simulink model "SmartAccess_20221026"  (R2022b)
settings: Solver=FixedStepDiscrete  StartTime=0.0  StopTime=10.0  RelTol=1e-3
undefined symbols (not defined in the file): AppPassthroughCommunicationOutputExternal, ApproachDetected, BasicUserInteractionFramework, GenericBackendMCPReceptions, GenericTelematicMCPReception, KeyPositionDetected, KeyProximityDetected, KeySearchRequest, KeyTrajectoryDetected, RequestDisplayCheckControl, RequestKeyPositionTracking, RequestKeyProximityTracking, RequestZa03ParkingandRemote, RequestZa06KlimaBasis, SendSmartAccessBackendData, SmartAccessEventNofitication, SmartAccessEventNotification, SmartAccessManageKey, SmartAccessTrackKey, SmartAccessVehicleUIControlAndStatus, StatusVehicleOccupantInformation, StopKeyPositionTracking, UpdateSmartAccessBackendData
settings Model: Creator=lcx19  LastModifiedBy=lcx19

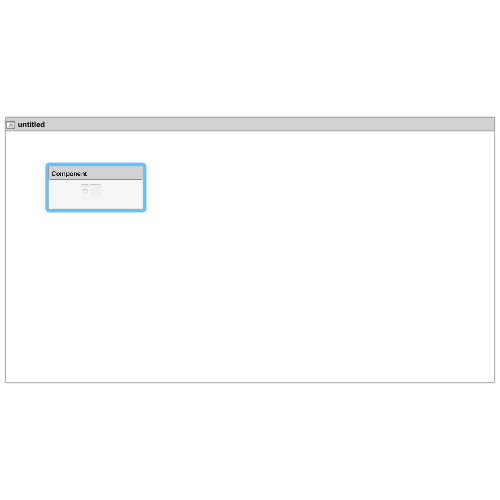
[thumbnail: Simulink's stored preview of the top-level diagram]
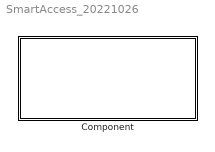
== system SmartAccess_20221026 ==
  Component : Subsystem
      settings: PortSchema="{\"entries\":[{\"content\":{\"headerSize\":26,\"margin\":15,\"minimumSpacing\":25,\"sides\":[{\"content\":{\"connectorIds\":[]},\"type\":\"ConnectorPlacement.EquallySpacedRectSide\",\"uuid\":\"a28210fe-8bcc-4966-9def-b490f12f7165\"},{\"content\":{\"connectorIds\":[],\"side\":\"RIGHT\"},\"type\":\"ConnectorPlacement.EquallySpacedRectSide\",\"uuid\":\"9429c510-dad9-436c-8408-75f9033cfc3b\"},{\"content\":{\"connectorIds\":[],\"side\":\"TOP\"},\"type\":\"ConnectorPlacement.EquallySpacedRectSide\",\"uuid\":\"a13e5907-bdbb-46b5-9334-9875d9723f49\"}]},\"type\":\"ConnectorPlacement.EquallySpacedConnector\",\"uuid\":\"ba0b5127-fa18-4541-84db-e1fe9f0ba6eb\"}],\"packageUris\":[\"http://schema.mathworks.com/mf0/Connector/R2020b\"],\"version\":\"1.0\"}"

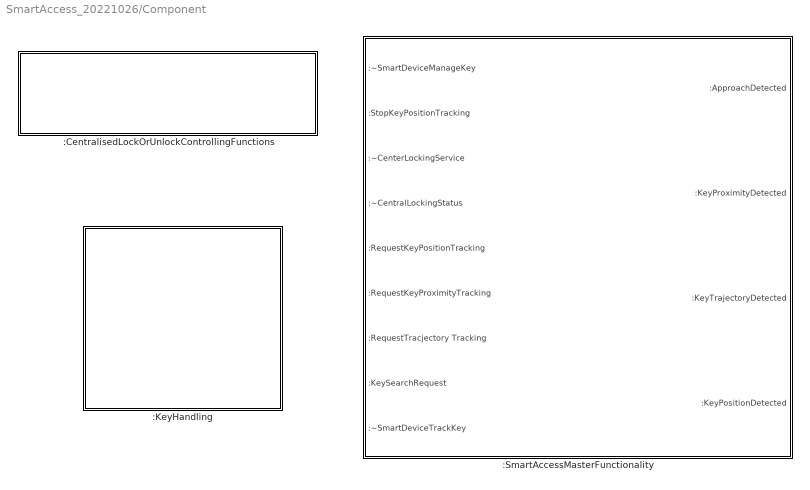
== system SmartAccess_20221026/Component ==
  :CentralisedLockOrUnlockControllingFunctions : Subsystem
      settings: PortSchema="{\"entries\":[{\"content\":{\"headerSize\":26,\"margin\":15,\"minimumSpacing\":25,\"sides\":[{\"content\":{\"connectorIds\":[]},\"type\":\"ConnectorPlacement.EquallySpacedRectSide\",\"uuid\":\"a28210fe-8bcc-4966-9def-b490f12f7165\"},{\"content\":{\"connectorIds\":[],\"side\":\"RIGHT\"},\"type\":\"ConnectorPlacement.EquallySpacedRectSide\",\"uuid\":\"9429c510-dad9-436c-8408-75f9033cfc3b\"},{\"content\":{\"connectorIds\":[],\"side\":\"TOP\"},\"type\":\"ConnectorPlacement.EquallySpacedRectSide\",\"uuid\":\"a13e5907-bdbb-46b5-9334-9875d9723f49\"}]},\"type\":\"ConnectorPlacement.EquallySpacedConnector\",\"uuid\":\"ba0b5127-fa18-4541-84db-e1fe9f0ba6eb\"}],\"packageUris\":[\"http://schema.mathworks.com/mf0/Connector/R2020b\"],\"version\":\"1.0\"}"
  :KeyHandling : Subsystem
      settings: PortSchema="{\"entries\":[{\"content\":{\"headerSize\":26,\"margin\":15,\"minimumSpacing\":25,\"sides\":[{\"content\":{\"connectorIds\":[]},\"type\":\"ConnectorPlacement.EquallySpacedRectSide\",\"uuid\":\"a28210fe-8bcc-4966-9def-b490f12f7165\"},{\"content\":{\"connectorIds\":[],\"side\":\"RIGHT\"},\"type\":\"ConnectorPlacement.EquallySpacedRectSide\",\"uuid\":\"9429c510-dad9-436c-8408-75f9033cfc3b\"},{\"content\":{\"connectorIds\":[],\"side\":\"TOP\"},\"type\":\"ConnectorPlacement.EquallySpacedRectSide\",\"uuid\":\"a13e5907-bdbb-46b5-9334-9875d9723f49\"}]},\"type\":\"ConnectorPlacement.EquallySpacedConnector\",\"uuid\":\"ba0b5127-fa18-4541-84db-e1fe9f0ba6eb\"}],\"packageUris\":[\"http://schema.mathworks.com/mf0/Connector/R2020b\"],\"version\":\"1.0\"}"
  :SmartAccessMasterFunctionality : Subsystem
      settings: PortSchema="{\"entries\":[{\"content\":{\"headerSize\":26,\"margin\":15,\"minimumSpacing\":25,\"sides\":[{\"content\":{\"connectorIds\":[\"In1\",\"In2\",\"Out1\",\"In3\",\"In4\",\"In5\",\"In6\",\"In7\",\"In8\"]},\"type\":\"ConnectorPlacement.EquallySpacedRectSide\",\"uuid\":\"a28210fe-8bcc-4966-9def-b490f12f7165\"},{\"content\":{\"connectorIds\":[\"Out2\",\"Out3\",\"Out4\",\"Out5\"],\"side\":\"RIGHT\"},\"type\":\"ConnectorPlacement.EquallySpacedRectSide\",\"uuid\":\"9429c510-dad9-436c-8408-75f9033cfc3b\"},{\"content\":{\"connectorIds\":[],\"side\":\"TOP\"},\"type\":\"ConnectorPlacement.EquallySpacedRectSide\",\"uuid\":\"a13e5907-bdbb-46b5-9334-9875d9723f49\"}]},\"type\":\"ConnectorPlacement.EquallySpacedConnector\",\"uuid\":\"ba0b5127-fa18-4541-84db-e1fe9f0ba6eb\"}],\"packageUris\":[\"http://schema.mathworks.com/mf0/Connector/R2020b\"],\"version\":\"1.0\"}"

== system SmartAccess_20221026/Component/:CentralisedLockOrUnlockControllingFunctions ==

== system SmartAccess_20221026/Component/:KeyHandling ==

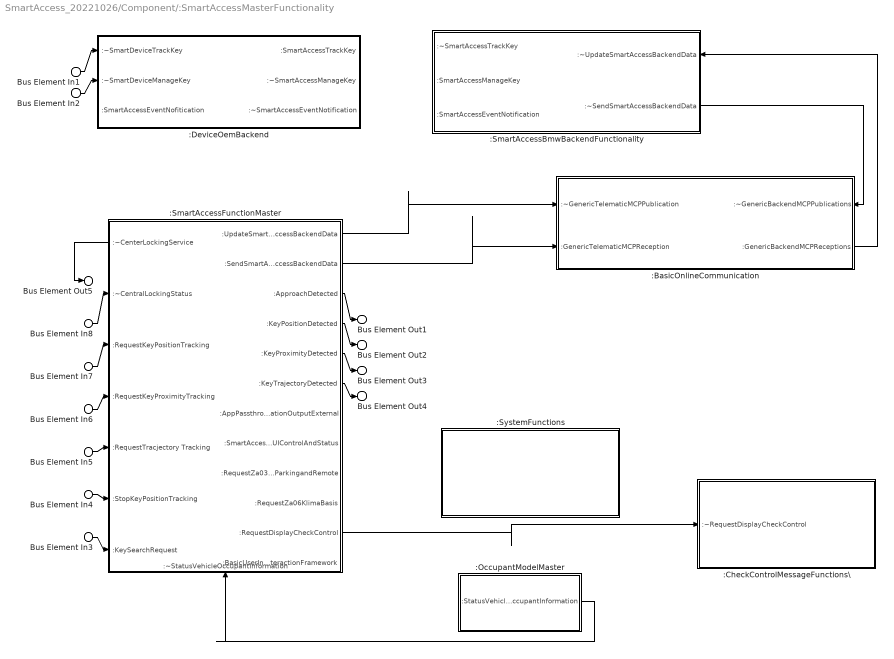
== system SmartAccess_20221026/Component/:SmartAccessMasterFunctionality ==
  Bus Element In2 : Inport  PortName=:~SmartDeviceManageKey
  Bus Element In4 : Inport  Port=2  PortName=:StopKeyPositionTracking
  Bus Element In8 : Inport  Port=3  PortName=:~CentralLockingStatus
  Bus Element In7 : Inport  Port=4  PortName=:RequestKeyPositionTracking
  Bus Element In6 : Inport  Port=5  PortName=:RequestKeyProximityTracking
  Bus Element In5 : Inport  Port=6  PortName=:RequestTracjectory Tracking
  Bus Element In3 : Inport  Port=7  PortName=:KeySearchRequest
  Bus Element In1 : Inport  Port=8  PortName=:~SmartDeviceTrackKey
  :BasicOnlineCommunication : Subsystem
      settings: PortSchema="{\"entries\":[{\"content\":{\"headerSize\":26,\"margin\":15,\"minimumSpacing\":25,\"sides\":[{\"content\":{\"connectorIds\":[\"In1\",\"In2\"]},\"type\":\"ConnectorPlacement.EquallySpacedRectSide\",\"uuid\":\"a28210fe-8bcc-4966-9def-b490f12f7165\"},{\"content\":{\"connectorIds\":[\"In3\",\"Out1\"],\"side\":\"RIGHT\"},\"type\":\"ConnectorPlacement.EquallySpacedRectSide\",\"uuid\":\"9429c510-dad9-436c-8408-75f9033cfc3b\"},{\"content\":{\"connectorIds\":[],\"side\":\"TOP\"},\"type\":\"ConnectorPlacement.EquallySpacedRectSide\",\"uuid\":\"a13e5907-bdbb-46b5-9334-9875d9723f49\"}]},\"type\":\"ConnectorPlacement.EquallySpacedConnector\",\"uuid\":\"ba0b5127-fa18-4541-84db-e1fe9f0ba6eb\"}],\"packageUris\":[\"http://schema.mathworks.com/mf0/Connector/R2020b\"],\"version\":\"1.0\"}"
  :CheckControlMessageFunctions\ : Subsystem
      settings: PortSchema="{\"entries\":[{\"content\":{\"headerSize\":26,\"margin\":15,\"minimumSpacing\":25,\"sides\":[{\"content\":{\"connectorIds\":[\"In1\"]},\"type\":\"ConnectorPlacement.EquallySpacedRectSide\",\"uuid\":\"a28210fe-8bcc-4966-9def-b490f12f7165\"},{\"content\":{\"connectorIds\":[],\"side\":\"RIGHT\"},\"type\":\"ConnectorPlacement.EquallySpacedRectSide\",\"uuid\":\"9429c510-dad9-436c-8408-75f9033cfc3b\"},{\"content\":{\"connectorIds\":[],\"side\":\"TOP\"},\"type\":\"ConnectorPlacement.EquallySpacedRectSide\",\"uuid\":\"a13e5907-bdbb-46b5-9334-9875d9723f49\"}]},\"type\":\"ConnectorPlacement.EquallySpacedConnector\",\"uuid\":\"ba0b5127-fa18-4541-84db-e1fe9f0ba6eb\"}],\"packageUris\":[\"http://schema.mathworks.com/mf0/Connector/R2020b\"],\"version\":\"1.0\"}"
  :DeviceOemBackend : Subsystem
      settings: PortSchema="{\"entries\":[{\"content\":{\"headerSize\":26,\"margin\":15,\"minimumSpacing\":25,\"sides\":[{\"content\":{\"connectorIds\":[\"In2\",\"In3\",\"In4\"]},\"type\":\"ConnectorPlacement.EquallySpacedRectSide\",\"uuid\":\"a28210fe-8bcc-4966-9def-b490f12f7165\"},{\"content\":{\"connectorIds\":[\"Out1\",\"Out2\",\"In1\"],\"side\":\"RIGHT\"},\"type\":\"ConnectorPlacement.EquallySpacedRectSide\",\"uuid\":\"9429c510-dad9-436c-8408-75f9033cfc3b\"},{\"content\":{\"connectorIds\":[],\"side\":\"TOP\"},\"type\":\"ConnectorPlacement.EquallySpacedRectSide\",\"uuid\":\"a13e5907-bdbb-46b5-9334-9875d9723f49\"}]},\"type\":\"ConnectorPlacement.EquallySpacedConnector\",\"uuid\":\"ba0b5127-fa18-4541-84db-e1fe9f0ba6eb\"}],\"packageUris\":[\"http://schema.mathworks.com/mf0/Connector/R2020b\"],\"version\":\"1.0\"}"
  :OccupantModelMaster : Subsystem
      settings: PortSchema="{\"entries\":[{\"content\":{\"headerSize\":26,\"margin\":15,\"minimumSpacing\":25,\"sides\":[{\"content\":{\"connectorIds\":[]},\"type\":\"ConnectorPlacement.EquallySpacedRectSide\",\"uuid\":\"a28210fe-8bcc-4966-9def-b490f12f7165\"},{\"content\":{\"connectorIds\":[\"Out1\"],\"side\":\"RIGHT\"},\"type\":\"ConnectorPlacement.EquallySpacedRectSide\",\"uuid\":\"9429c510-dad9-436c-8408-75f9033cfc3b\"},{\"content\":{\"connectorIds\":[],\"side\":\"TOP\"},\"type\":\"ConnectorPlacement.EquallySpacedRectSide\",\"uuid\":\"a13e5907-bdbb-46b5-9334-9875d9723f49\"}]},\"type\":\"ConnectorPlacement.EquallySpacedConnector\",\"uuid\":\"ba0b5127-fa18-4541-84db-e1fe9f0ba6eb\"}],\"packageUris\":[\"http://schema.mathworks.com/mf0/Connector/R2020b\"],\"version\":\"1.0\"}"
  :SmartAccessBmwBackendFunctionality : Subsystem
      settings: PortSchema="{\"entries\":[{\"content\":{\"headerSize\":26,\"margin\":15,\"minimumSpacing\":25,\"sides\":[{\"content\":{\"connectorIds\":[\"In2\",\"In3\",\"Out2\"]},\"type\":\"ConnectorPlacement.EquallySpacedRectSide\",\"uuid\":\"a28210fe-8bcc-4966-9def-b490f12f7165\"},{\"content\":{\"connectorIds\":[\"In1\",\"Out1\"],\"side\":\"RIGHT\"},\"type\":\"ConnectorPlacement.EquallySpacedRectSide\",\"uuid\":\"9429c510-dad9-436c-8408-75f9033cfc3b\"},{\"content\":{\"connectorIds\":[],\"side\":\"TOP\"},\"type\":\"ConnectorPlacement.EquallySpacedRectSide\",\"uuid\":\"a13e5907-bdbb-46b5-9334-9875d9723f49\"}]},\"type\":\"ConnectorPlacement.EquallySpacedConnector\",\"uuid\":\"ba0b5127-fa18-4541-84db-e1fe9f0ba6eb\"}],\"packageUris\":[\"http://schema.mathworks.com/mf0/Connector/R2020b\"],\"version\":\"1.0\"}"
  :SmartAccessFunctionMaster : Subsystem
      settings: PortSchema="{\"entries\":[{\"content\":{\"headerSize\":26,\"margin\":15,\"minimumSpacing\":25,\"sides\":[{\"content\":{\"connectorIds\":[\"Out1\",\"In1\",\"In2\",\"In3\",\"In4\",\"In5\",\"In6\"]},\"type\":\"ConnectorPlacement.EquallySpacedRectSide\",\"uuid\":\"a28210fe-8bcc-4966-9def-b490f12f7165\"},{\"content\":{\"connectorIds\":[\"Out2\",\"Out3\",\"Out4\",\"Out5\",\"Out6\",\"Out7\",\"Out8\",\"Out9\",\"Out10\",\"Out11\",\"Out12\",\"Out13\"],\"side\":\"RIGHT\"},\"type\":\"ConnectorPlacement.EquallySpacedRectSide\",\"uuid\":\"9429c510-dad9-436c-8408-75f9033cfc3b\"},{\"content\":{\"connectorIds\":[],\"side\":\"TOP\"},\"type\":\"ConnectorPlacement.EquallySpacedRectSide\",\"uuid\":\"a13e5907-bdbb-46b5-9334-9875d9723f49\"},{\"content\":{\"connectorIds\":[\"In7\"],\"side\":\"BOTTOM\"},\"type\":\"ConnectorPlacement.EquallySpacedRectSide\",\"uuid\":\"de40a1c8-ef0d-4a2a-ba46-2e2a24800d7b\"}]},\"type\":\"ConnectorPlacement.EquallySpacedConnector\",\"uuid\":\"ba0b5127-fa18-4541-84db-e1fe9f0ba6eb\"}],\"packageUris\":[\"http://schema.mathworks.com/mf0/Connector/R2020b\"],\"version\":\"1.0\"}"
  :SystemFunctions : Subsystem
      settings: PortSchema="{\"entries\":[{\"content\":{\"headerSize\":26,\"margin\":15,\"minimumSpacing\":25,\"sides\":[{\"content\":{\"connectorIds\":[]},\"type\":\"ConnectorPlacement.EquallySpacedRectSide\",\"uuid\":\"a28210fe-8bcc-4966-9def-b490f12f7165\"},{\"content\":{\"connectorIds\":[],\"side\":\"RIGHT\"},\"type\":\"ConnectorPlacement.EquallySpacedRectSide\",\"uuid\":\"9429c510-dad9-436c-8408-75f9033cfc3b\"},{\"content\":{\"connectorIds\":[],\"side\":\"TOP\"},\"type\":\"ConnectorPlacement.EquallySpacedRectSide\",\"uuid\":\"a13e5907-bdbb-46b5-9334-9875d9723f49\"}]},\"type\":\"ConnectorPlacement.EquallySpacedConnector\",\"uuid\":\"ba0b5127-fa18-4541-84db-e1fe9f0ba6eb\"}],\"packageUris\":[\"http://schema.mathworks.com/mf0/Connector/R2020b\"],\"version\":\"1.0\"}"
  Bus Element Out5 : Outport  PortName=:~CenterLockingService
  Bus Element Out1 : Outport  Port=2  PortName=:ApproachDetected
  Bus Element Out3 : Outport  Port=3  PortName=:KeyProximityDetected
  Bus Element Out4 : Outport  Port=4  PortName=:KeyTrajectoryDetected
  Bus Element Out2 : Outport  Port=5  PortName=:KeyPositionDetected
  wires:
  Bus Element In1/1 -> :DeviceOemBackend/2(:~SmartDeviceTrackKey)
  Bus Element In2/1 -> :DeviceOemBackend/3(:~SmartDeviceManageKey)
  :SmartAccessBmwBackendFunctionality/1(:~SendSmartAccessBackendData) -> :BasicOnlineCommunication/3(:~GenericBackendMCPPublications)
  :BasicOnlineCommunication/1(:GenericBackendMCPReceptions) -> :SmartAccessBmwBackendFunctionality/1(:~UpdateSmartAccessBackendData)
  :SmartAccessFunctionMaster/2(:UpdateSmartAccessBackendData) -> :BasicOnlineCommunication/1(:~GenericTelematicMCPPublication)
  :SmartAccessFunctionMaster/3(:SendSmartAccessBackendData) -> :BasicOnlineCommunication/2(:GenericTelematicMCPReception)
  :SmartAccessFunctionMaster/4(:ApproachDetected) -> Bus Element Out1/1
  :SmartAccessFunctionMaster/5(:KeyPositionDetected) -> Bus Element Out2/1
  :SmartAccessFunctionMaster/6(:KeyProximityDetected) -> Bus Element Out3/1
  :SmartAccessFunctionMaster/7(:KeyTrajectoryDetected) -> Bus Element Out4/1
  :SmartAccessFunctionMaster/12(:RequestDisplayCheckControl) -> :CheckControlMessageFunctions\/1(:~RequestDisplayCheckControl)
  :OccupantModelMaster/1(:StatusVehicleOccupantInformation) -> :SmartAccessFunctionMaster/7(:~StatusVehicleOccupantInformation)
  Bus Element In3/1 -> :SmartAccessFunctionMaster/6(:KeySearchRequest)
  Bus Element In4/1 -> :SmartAccessFunctionMaster/5(:StopKeyPositionTracking)
  Bus Element In5/1 -> :SmartAccessFunctionMaster/4(:RequestTracjectory Tracking)
  :SmartAccessFunctionMaster/1(:~CenterLockingService) -> Bus Element Out5/1
  Bus Element In6/1 -> :SmartAccessFunctionMaster/3(:RequestKeyProximityTracking)
  Bus Element In7/1 -> :SmartAccessFunctionMaster/2(:RequestKeyPositionTracking)
  Bus Element In8/1 -> :SmartAccessFunctionMaster/1(:~CentralLockingStatus)

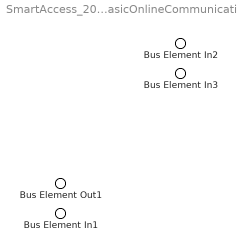
== system SmartAccess_20221026/Component/:SmartAccessMasterFunctionality/:BasicOnlineCommunication ==
  Bus Element In2 : Inport  PortName=:~GenericTelematicMCPPublication
  Bus Element In3 : Inport  Port=2  PortName=:GenericTelematicMCPReception
  Bus Element In1 : Inport  Port=3  PortName=:~GenericBackendMCPPublications
  Bus Element Out1 : Outport  PortName=:GenericBackendMCPReceptions

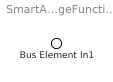
== system SmartAccess_20221026/Component/:SmartAccessMasterFunctionality/:CheckControlMessageFunctions\ ==
  Bus Element In1 : Inport  PortName=:~RequestDisplayCheckControl

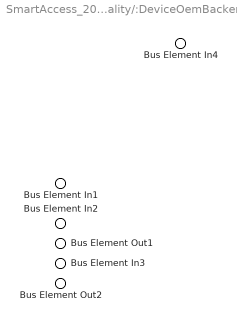
== system SmartAccess_20221026/Component/:SmartAccessMasterFunctionality/:DeviceOemBackend ==
  Bus Element In4 : Inport  PortName=:~SmartAccessEventNotification
  Bus Element In1 : Inport  Port=2  PortName=:~SmartDeviceTrackKey
  Bus Element In2 : Inport  Port=3  PortName=:~SmartDeviceManageKey
  Bus Element In3 : Inport  Port=4  PortName=:SmartAccessEventNofitication
  Bus Element Out1 : Outport  PortName=:SmartAccessTrackKey
  Bus Element Out2 : Outport  Port=2  PortName=:~SmartAccessManageKey

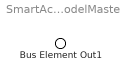
== system SmartAccess_20221026/Component/:SmartAccessMasterFunctionality/:OccupantModelMaster ==
  Bus Element Out1 : Outport  PortName=:StatusVehicleOccupantInformation

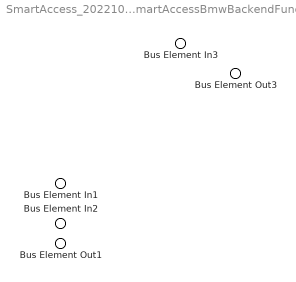
== system SmartAccess_20221026/Component/:SmartAccessMasterFunctionality/:SmartAccessBmwBackendFunctionality ==
  Bus Element In3 : Inport  PortName=:~UpdateSmartAccessBackendData
  Bus Element In1 : Inport  Port=2  PortName=:~SmartAccessTrackKey
  Bus Element In2 : Inport  Port=3  PortName=:SmartAccessManageKey
  Bus Element Out3 : Outport  PortName=:~SendSmartAccessBackendData
  Bus Element Out1 : Outport  Port=2  PortName=:SmartAccessEventNotification

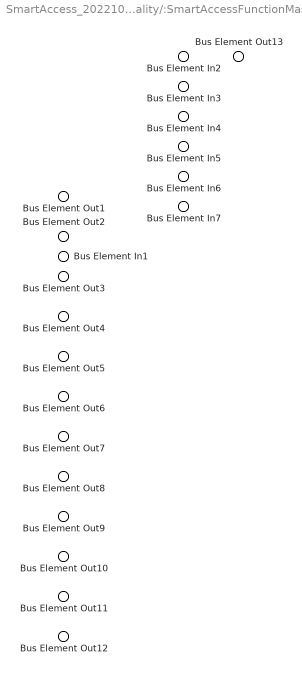
== system SmartAccess_20221026/Component/:SmartAccessMasterFunctionality/:SmartAccessFunctionMaster ==
  Bus Element In7 : Inport  PortName=:~CentralLockingStatus
  Bus Element In6 : Inport  Port=2  PortName=:RequestKeyPositionTracking
  Bus Element In5 : Inport  Port=3  PortName=:RequestKeyProximityTracking
  Bus Element In4 : Inport  Port=4  PortName=:RequestTracjectory Tracking
  Bus Element In3 : Inport  Port=5  PortName=:StopKeyPositionTracking
  Bus Element In2 : Inport  Port=6  PortName=:KeySearchRequest
  Bus Element In1 : Inport  Port=7  PortName=:~StatusVehicleOccupantInformation
  Bus Element Out13 : Outport  PortName=:~CenterLockingService
  Bus Element Out1 : Outport  Port=2  PortName=:UpdateSmartAccessBackendData
  Bus Element Out2 : Outport  Port=3  PortName=:SendSmartAccessBackendData
  Bus Element Out3 : Outport  Port=4  PortName=:ApproachDetected
  Bus Element Out4 : Outport  Port=5  PortName=:KeyPositionDetected
  Bus Element Out5 : Outport  Port=6  PortName=:KeyProximityDetected
  Bus Element Out6 : Outport  Port=7  PortName=:KeyTrajectoryDetected
  Bus Element Out7 : Outport  Port=8  PortName=:AppPassthroughCommunicationOutputExternal
  Bus Element Out8 : Outport  Port=9  PortName=:SmartAccessVehicleUIControlAndStatus
  Bus Element Out9 : Outport  Port=10  PortName=:RequestZa03ParkingandRemote
  Bus Element Out10 : Outport  Port=11  PortName=:RequestZa06KlimaBasis
  Bus Element Out11 : Outport  Port=12  PortName=:RequestDisplayCheckControl
  Bus Element Out12 : Outport  Port=13  PortName=:BasicUserInteractionFramework

== system SmartAccess_20221026/Component/:SmartAccessMasterFunctionality/:SystemFunctions ==
